simulink model "untitled5"  (R2024b)
settings: Solver=FixedStepAuto  StartTime=0.0  StopTime=totalTime  FixedStep=deltaT  RelTol=1e-3
values from neighbouring files (symbols this model uses):
  A = [0 1 0 0 ... (first row only)    [XYZregulators.m]    (also in XYZregulators_try_with_simulink.m; maticeABC.m = [0 0 0 1 0 0 0 0  0 0; rir.m = [0  0  0  1  0  0  0  0  0  0                 0             )
  B = [0 0 ... (first row only)    [XYZregulators.m]    (also in XYZregulators_try_with_simulink.m; maticeABC.m = [0 0 0 0; rir.m = [0     0     0     0)
  C = [1 0 0 0]    [XYZregulators.m]    (also in XYZregulators_try_with_simulink.m; maticeABC.m = [1 0 0 0 0 0 0 0 0 0; rir.m = [1  0  0  0  0  0  0  0  0  0  0  0)
undefined symbols (not defined in the file or in its folder): den, num
settings Model: Creator=matys  LastModifiedBy=Michael
settings RTWCC: GPUComputeCapability=3.5

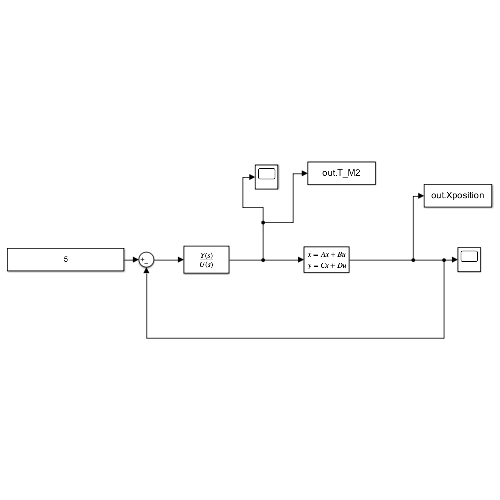
[thumbnail: Simulink's stored preview of the top-level diagram]
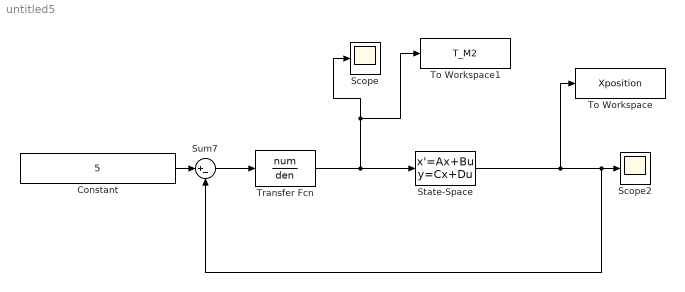
== system untitled5 ==
  Constant : Constant  Value=5
  Scope : Scope
  Scope2 : Scope
  State-Space : StateSpace  A=A  B=B  C=C  D=zeros(1,2)  InitialCondition=0
  Sum7 : Sum  Inputs=|+-
  To Workspace : ToWorkspace  VariableName=Xposition  SaveFormat=Timeseries  SampleTime=-1
  To Workspace1 : ToWorkspace  VariableName=T_M2  SaveFormat=Timeseries  SampleTime=-1
  Transfer Fcn : TransferFcn  Numerator=num  Denominator=den
  wires:
  Sum7/1 -> Transfer Fcn/1
  Constant/1 -> Sum7/1
  State-Space/1 -> To Workspace/1, Sum7/2, Scope2/1
  Transfer Fcn/1 -> State-Space/1, To Workspace1/1, Scope/1
